simulink model "kundur_no_pss_all_methodes"  (R2023a)
settings: Solver=ode23tb  StartTime=0.0  StopTime=20  MaxStep=1/60  RelTol=1e-4  EnableMultiTasking=on
InitFcn:
  | N=200;
  | Ts=1/60;
undefined symbols (not defined in the file or in its folder): D1, Delta
libraries: spsLoadFlowBusLib x6, spsThreePhaseParallelRLCLoadLib x5, spsThreePhasePISectionLineLib x4, spsSynchronousMachinepuStandardLib x4, spsThreePhaseTransformerTwoWindingsLib x4, spsDistributedParametersLineLib x3, spsThreePhaseVIMeasurementLib x2, spsSequenceAnalyzerPhasorLib x2, spsThreePhaseBreakerLib x1, spsPower3phPhasorLib x1, spspowerguiLib x1
Description:
  | Copyright 2008-2015 The MathWorks, Inc.
settings Model: ExtModeTrigMode=oneshot  Creator=MathWorks  LastModifiedBy=felixmaldonado
settings SolverCC: AlgebraicLoopSolver=TrustRegion
settings DataIOCC: SaveFormat=Array  SignalLoggingSaveFormat=ModelDataLogs  SaveOutput=off  SaveTime=off  ReturnWorkspaceOutputs=off  TimeSaveName=t  SignalLoggingName=sigsOut
settings OptimizationCC: BlockReduction=off  BooleanDataType=off  ExpressionDepthLimit=2147483647  InitFltsAndDblsToZero=on  LifeSpan=inf
settings DebuggingCC: UnderspecifiedInitializationDetection=Classic  MergeDetectMultiDrivingBlocksExec=none  SignalResolutionControl=TryResolveAllWithWarning  MultiTaskDSMMsg=warning  MultiTaskCondExecSysMsg=none  FcnCallInpInsideContextMsg=warning  UnconnectedInputMsg=warning  UnconnectedLineMsg=warning  StateNameClashWarn=warning  SFUnexpectedBacktrackingDiag=warning  SFNoUnconditionalDefaultTransitionDiag=warning  SFExecutionAtInitializationDiag=none  ArithmeticOperatorsInVariantConditions=warning
settings HardwareCC: ProdBitPerPointer=32  ProdBitPerSizeT=32  ProdBitPerPtrDiffT=32  ProdLargestAtomicFloat=None  ProdIntDivRoundTo=Undefined  ProdEndianess=Unspecified  ProdWordSize=32  ProdHWDeviceType=32-bit Generic  TargetUnknown=on
settings ModelReferenceCC: PropagateSignalLabelsOutOfModel=off
settings SFSimCC: SimUseLocalCustomCode=off  CustomCodeUndefinedFunction=UseInterfaceOnly
settings RTWCC: RTWUseLocalCustomCode=off
settings CodeAppCC: StateflowObjectComments=on
settings GRTTargetCC: TargetLangStandard=C89/C90 (ANSI)  CombineOutputUpdateFcns=off  GRTInterface=on
settings ConfigComp: CovMetricSettings=dw  CovSaveCumulativeToWorkspaceVar=on  CovSaveSingleToWorkspaceVar=on  CovExternalEMLEnable=off  CovSFcnEnable=off
settings SimscapeCC: SimscapeNormalizeSystem=off

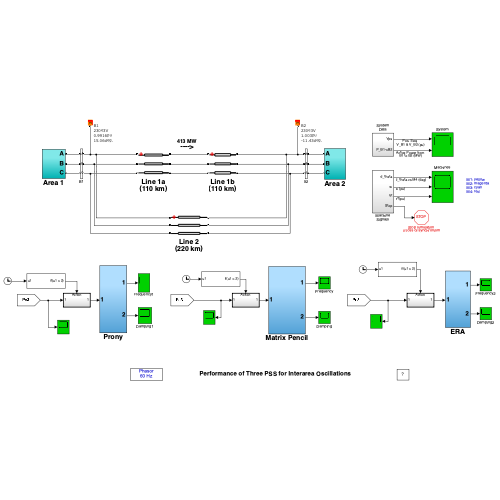
[thumbnail: Simulink's stored preview of the top-level diagram]
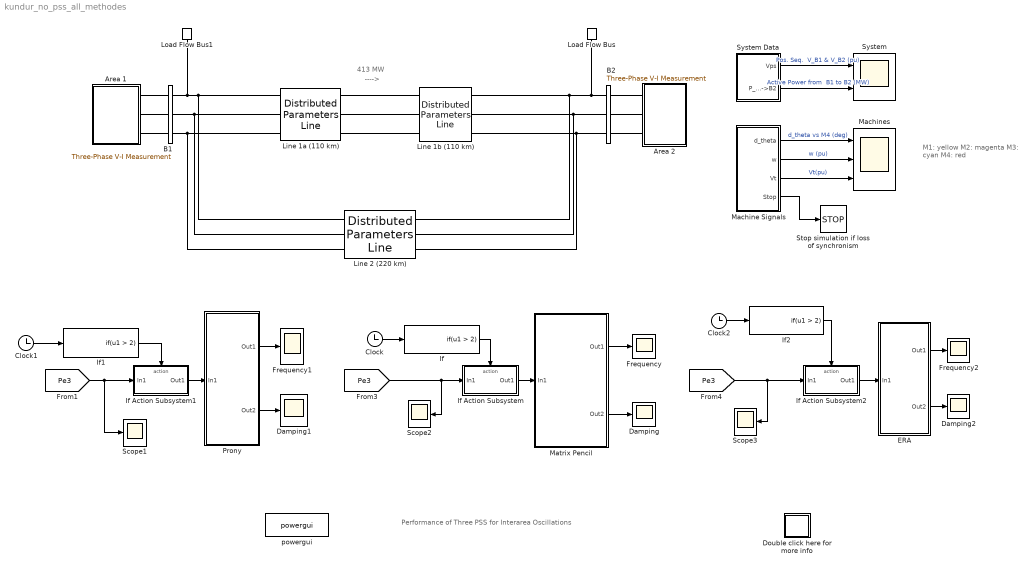
== system kundur_no_pss_all_methodes ==
  note: Performance of Three PSS for Interarea Oscillations
  note: M1: yellow
      | M2: magenta
      | M3: cyan
      | M4: red
  note: ---->
  note: 413 MW
  Area 1 : Subsystem
  Area 2 : Subsystem
  B1 : spsThreePhaseVIMeasurementLib/Three-Phase V-I Measurement  VoltageMeasurement=phase-to-ground  SetLabelV=on  LabelV=Vabc_B1  Vpu=off  VpuLL=off  CurrentMeasurement=yes  SetLabelI=on  LabelI=Iabc_B1  Ipu=off  Pbase=100e6  Vbase=500e3  OutputType=Complex  PhasorSimulation=on  PSBequivalent=0
  B2 : spsThreePhaseVIMeasurementLib/Three-Phase V-I Measurement  VoltageMeasurement=phase-to-ground  SetLabelV=on  LabelV=Vabc_B2  Vpu=off  VpuLL=off  CurrentMeasurement=yes  SetLabelI=on  LabelI=Iabc_B2  Ipu=off  Pbase=100e6  Vbase=500e3  OutputType=Complex  PhasorSimulation=on  PSBequivalent=0
  Clock : Clock
  Clock1 : Clock
  Clock2 : Clock
  Damping : Scope
  Damping1 : Scope
  Damping2 : Scope
  Double click here for more info : Subsystem
      settings: OpenFcn=showdemo(bdroot(gcb))
      mask Display: disp('?')
  ERA : Subsystem
  Frequency : Scope
  Frequency1 : Scope
  Frequency2 : Scope
  If : If  IfExpression=u1 > 2  ShowElse=off
  If Action Subsystem : Subsystem  TreatAsAtomicUnit=on
  If Action Subsystem1 : Subsystem  TreatAsAtomicUnit=on
  If Action Subsystem2 : Subsystem  TreatAsAtomicUnit=on
  If1 : If  IfExpression=u1 > 2  ShowElse=off
  If2 : If  IfExpression=u1 > 2  ShowElse=off
  Line 1a (110 km) : spsDistributedParametersLineLib/Distributed Parameters Line  Phases=3  Length=110  Frequency=60  Resistance=[0.0001*529 1.61]  Inductance=[0.001*529/(377) 0.0061]  Capacitance=[0.00175/529/(377) 5.2489e-9]  x1=[3.8639158388023e-08 228065.282846779 228065.232417196;376.991118430775 376.991118430775 376.991118430775;-0.600540727316574 0.641001708190165 -0.929792189501776]  x2=[2.61662140985057e-08 225633.072942765 225632.837043247;376.991118430775 376.991118430775 376.991118430775;-0.986420545168886 0.407422059296571 -1.16337164754703]  x3=[2.2632718889879e-11 336.03871645381 336.037634042508;376.991118430775 376.991118430775 376.991118430775;1.8256601366186 -2.54731502272154 2.16506718382181]  x4=[7.36776449333454e-11 1450.99138096572 1450.98995609566;376.991118430775 376.991118430775 376.991118430775;-1.01301435290975 0.484705984236178 -1.08608998759577]  x5=0.000622431770558027  V1=ones(3,3)  V2=ones(3,3)  I1=ones(3,3)  I2=ones(3,3)  nHarmo=1  Measurements=None  Decoupling=off  VsMag0=0  VrMag0=0  VsAngle0=0  VrAngle0=0  IsMag0=0  IrMag0=0  IsAngle0=0  IrAngle0=0
      settings: AttributesFormatString=\n  LibrarySourceBlock=sps_lib/Power Grid Elements/Distributed Parameters Line
  Line 1b (110 km) : spsDistributedParametersLineLib/Distributed Parameters Line  Phases=3  Length=110  Frequency=60  Resistance=[0.0001*529 1.61]  Inductance=[0.001*529/(377) 0.0061]  Capacitance=[0.00175/529/(377) 5.2489e-9]  x1=[2.61662140985057e-08 225633.072942765 225632.837043247;376.991118430775 376.991118430775 376.991118430775;-0.986420545168886 0.407422059296571 -1.16337164754703]  x2=[1.96331439687636e-08 230635.983486102 230635.554670201;376.991118430775 376.991118430775 376.991118430775;-1.70223885434449 0.178613473681849 -1.39218042790549]  x3=[2.98939585655011e-11 348.890847759972 348.889760478068;376.991118430775 376.991118430775 376.991118430775;2.05678749014555 -2.40728630159656 2.30509610560278]  x4=[6.51521319057991e-11 1438.08029667253 1438.07888403635;376.991118430775 376.991118430775 376.991118430775;-1.27922422756789 0.338636937194732 -1.2321590219245]  x5=0.000622431770558027  V1=ones(3,3)  V2=ones(3,3)  I1=ones(3,3)  I2=ones(3,3)  nHarmo=1  Measurements=None  Decoupling=off  VsMag0=0  VrMag0=0  VsAngle0=0  VrAngle0=0  IsMag0=0  IrMag0=0  IsAngle0=0  IrAngle0=0
      settings: AttributesFormatString=\n  LibrarySourceBlock=sps_lib/Power Grid Elements/Distributed Parameters Line
  Line 2 (220 km) : spsDistributedParametersLineLib/Distributed Parameters Line  Phases=3  Length=220  Frequency=60  Resistance=[0.0001*529 1.61]  Inductance=[0.001*529/(377) 0.0061]  Capacitance=[0.00175/529/(377) 5.2489e-9]  x1=[3.8639158388023e-08 228065.282846779 228065.232417196;376.991118430775 376.991118430775 376.991118430775;-0.835191976646093 0.49548881423357 -1.07530508345837]  x2=[1.96331439687636e-08 230635.983486102 230635.554670201;376.991118430775 376.991118430775 376.991118430775;-1.936890103674 0.0331005797252549 -1.53769332186209]  x3=[2.18539779503067e-11 335.641578515064 335.640503974824;376.991118430775 376.991118430775 376.991118430775;1.57451462094119 -2.69325063508951 2.01913162677061]  x4=[5.95777091396547e-11 1425.67040358948 1425.6690039208;376.991118430775 376.991118430775 376.991118430775;-1.49093562018794 0.193193498573398 -1.37760246372871]  x5=0.00124486354111605  V1=ones(3,3)  V2=ones(3,3)  I1=ones(3,3)  I2=ones(3,3)  nHarmo=1  Measurements=None  Decoupling=off  VsMag0=0  VrMag0=0  VsAngle0=0  VrAngle0=0  IsMag0=0  IrMag0=0  IsAngle0=0  IrAngle0=0
      settings: AttributesFormatString=\n  LibrarySourceBlock=sps_lib/Power Grid Elements/Distributed Parameters Line
  Load Flow Bus : spsLoadFlowBusLib/Load Flow Bus  LConnTagsString=a  Phases=single  Connectors=on one side  ID=B2  Vbase=230e3  Vref=1  Vangle=0  VLF=1.003  VLFb=1  VLFc=1  angleLF=-11.43  angleLFb=0  angleLFc=0
      settings: AttributesFormatString=%<ID>\n%<Vbase>V\n%<VLF>pu\n%<angleLF>deg.
  Load Flow Bus1 : spsLoadFlowBusLib/Load Flow Bus  LConnTagsString=a  Phases=single  Connectors=on one side  ID=B1  Vbase=230e3  Vref=1  Vangle=0  VLF=0.9916  VLFb=1  VLFc=1  angleLF=15.06  angleLFb=0  angleLFc=0
      settings: AttributesFormatString=%<ID>\n%<Vbase>V\n%<VLF>pu\n%<angleLF>deg.
  Machine Signals : Subsystem
  Machines : Scope  NumInputPorts=3
  Matrix Pencil : Subsystem
  Prony : Subsystem
  Scope1 : Scope
  Scope2 : Scope
  Scope3 : Scope
  Stop simulation if loss of synchronism : Stop
  System : Scope  NumInputPorts=2
  System Data : Subsystem
  powergui : spspowerguiLib/powergui  Priority=2  SimulationMode=Phasor  SampleTime=0  frequency=60  Iterations=50  frequencyindice=60  Pbase=100e6  ErrMax=0.0001  UnitsV=kV  UnitsW=MW  buscounter=0  FunctionMessages=off  echomessages=on  EnableUseOfTLC=off  CurrentSourceSwitches=off  DisableSnubberDevices=off  DisableRonSwitches=off  DisableVfSwitches=off  DisplayEquations=off  AutomaticDiscreteSolvers=off  SolverType=Tustin  Interpol=off  ExternalGateDelay=off  methode=off  Ts=0  x0status=steady  SPID=off  SwTol=0  HookPort=off  NonlinearTolerance=1e-4  nMaxIteration=100  ContinueOnMaxIteration=off  RestoreLinks=warning  ResistiveCurrentMeasurement=off  Frange=logspace(0,3,50)  Ylog=off  Xlog=off  ShowGrid=off  save=off  variable=ZData  structure=0  ZoomFFT=on  StartTime=0.0  cycles=1  DisplayStyle=1  fundamental=60  FreqAxis=off  MaxFrequency=1000  frequencyindicesteady=1  RmsSteady=1  display=off
  wires:
  Machine Signals/1(d_theta) -> Machines/1  "d_theta vs M4 (deg)"
  Machine Signals/2(w) -> Machines/2  "w (pu)"
  Machine Signals/3(Vt) -> Machines/3  "Vt(pu)"
  Machine Signals/4(Stop) -> Stop simulation if loss of synchronism/1
  System Data/1(Vps) -> System/1  "Pos. Seq.  V_B1 & V_B2 (pu)"
  System Data/2(P_B1->B2) -> System/2  "Active Power from  B1 to B2 (MW)"
  Clock/1 -> If/1
  If/1 -> If Action Subsystem/Action
  If Action Subsystem/1(Out1) -> Matrix Pencil/1(In1)
  [Pe3] -> Scope2/1, If Action Subsystem/1(In1)
  Matrix Pencil/1(Out1) -> Frequency/1
  Matrix Pencil/2(Out2) -> Damping/1
  Clock1/1 -> If1/1
  If1/1 -> If Action Subsystem1/Action
  If Action Subsystem1/1(Out1) -> Prony/1(In1)
  Prony/1(Out1) -> Frequency1/1
  Prony/2(Out2) -> Damping1/1
  [Pe3] -> Scope1/1, If Action Subsystem1/1(In1)
  Clock2/1 -> If2/1
  If2/1 -> If Action Subsystem2/Action
  If Action Subsystem2/1(Out1) -> ERA/1(In1)
  [Pe3] -> Scope3/1, If Action Subsystem2/1(In1)
  ERA/1(Out1) -> Frequency2/1
  ERA/2(Out2) -> Damping2/1
  connections:
  B1/RConn1 -- Line 1a (110 km)/LConn1 -- Line 2 (220 km)/LConn1 -- Load Flow Bus1/LConn1
  B1/RConn3 -- Line 1a (110 km)/LConn3 -- Line 2 (220 km)/LConn3
  Line 1b (110 km)/LConn1 -- Line 1a (110 km)/RConn1
  Line 1b (110 km)/LConn2 -- Line 1a (110 km)/RConn2
  Line 1a (110 km)/RConn3 -- Line 1b (110 km)/LConn3
  B2/LConn2 -- Line 1b (110 km)/RConn2 -- Line 2 (220 km)/RConn2
  Area 1/RConn2 -- B1/LConn2
  Area 1/RConn1 -- B1/LConn1
  Area 1/RConn3 -- B1/LConn3
  B1/RConn2 -- Line 1a (110 km)/LConn2 -- Line 2 (220 km)/LConn2
  B2/RConn2 -- Area 2/LConn2
  B2/RConn1 -- Area 2/LConn1
  B2/RConn3 -- Area 2/LConn3
  B2/LConn1 -- Line 1b (110 km)/RConn1 -- Line 2 (220 km)/RConn1 -- Load Flow Bus/LConn1
  B2/LConn3 -- Line 1b (110 km)/RConn3 -- Line 2 (220 km)/RConn3

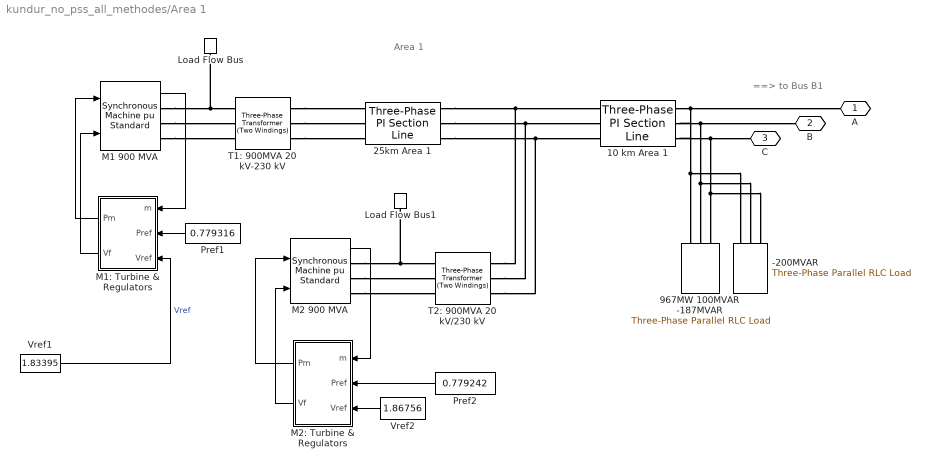
== system kundur_no_pss_all_methodes/Area 1 ==
  note: Area 1
  note: ==> to Bus B1
  -200MVAR : spsThreePhaseParallelRLCLoadLib/Three-Phase Parallel RLC Load  LConnTagsString=A|B|C  Configuration=Y (grounded)  NominalVoltage=230e3  Vabc=[1e3 1e3 1e3]  Vabcp=[1e3 1e3 1e3]  NominalFrequency=60  UnbalancedPower=off  ActivePower=0  InductivePower=0  CapacitivePower=200e6  Pabc=[10e3 9e3 11e3]  QLabc=[100 90 110]  QCabc=[100 90 110]  Pabcp=[10e3 9e3 11e3]  QLabcp=[100 90 110]  QCabcp=[100 90 110]  Measurements=None  LoadType=constant Z
  10 km Area 1 : spsThreePhasePISectionLineLib/Three-Phase PI Section Line  LConnTagsString=a|b|c  RConnTagsString=A|B|C  Length=10  Frequency=60  Resistances=[0.0001*529 1.61]  Inductances=[0.001*529/(377) 0.0061]  Capacitances=[0.00175/529/(377) 5.2489e-9]
  25km Area 1 : spsThreePhasePISectionLineLib/Three-Phase PI Section Line  LConnTagsString=a|b|c  RConnTagsString=A|B|C  Length=25  Frequency=60  Resistances=[0.0001*529 1.61]  Inductances=[0.001*529/(377) 0.0061]  Capacitances=[0.00175/529/(377) 5.2489e-9]
  967MW 100MVAR -187MVAR : spsThreePhaseParallelRLCLoadLib/Three-Phase Parallel RLC Load  LConnTagsString=A|B|C  Configuration=Y (grounded)  NominalVoltage=230e3  Vabc=[1e3 1e3 1e3]  Vabcp=[1e3 1e3 1e3]  NominalFrequency=60  UnbalancedPower=off  ActivePower=967000000  InductivePower=100e6  CapacitivePower=187e6  Pabc=[10e3 9e3 11e3]  QLabc=[100 90 110]  QCabc=[100 90 110]  Pabcp=[10e3 9e3 11e3]  QLabcp=[100 90 110]  QCabcp=[100 90 110]  Measurements=None  LoadType=constant Z
  Load Flow Bus : spsLoadFlowBusLib/Load Flow Bus  LConnTagsString=a  Phases=single  Connectors=on one side  ID=M1_Area1  Vbase=20e3  Vref=1  Vangle=0  VLF=1  VLFb=1  VLFc=1  angleLF=10.22  angleLFb=0  angleLFc=0
      settings: AttributesFormatString=%<ID>\n%<Vbase>V\n%<VLF>pu\n%<angleLF>deg.
  Load Flow Bus1 : spsLoadFlowBusLib/Load Flow Bus  LConnTagsString=a  Phases=single  Connectors=on one side  ID=M2_Area1  Vbase=20e3  Vref=1  Vangle=0  VLF=1  VLFb=1  VLFc=1  angleLF=0  angleLFb=0  angleLFc=0
      settings: AttributesFormatString=%<ID>\n%<Vbase>V\n%<VLF>pu\n%<angleLF>deg.
  M1 900 MVA : spsSynchronousMachinepuStandardLib/Synchronous Machine pu Standard  PresetModel=No  MechanicalLoad=Mechanical power Pm  ShowDetailedParameters=on  RotorType=Round  Units=per unit standard parameters  MeasurementBus=off  NominalParameters="[900E6  20000   60 ]"  Reactances1=[1.8 .3 .25 1.7 .55 .25 .2]  Reactances2=[ 1.305, 0.296, 0.252, 0.474, 0.243, 0.18 ]  dAxisTimeConstants=Open-circuit  qAxisTimeConstants=Open-circuit  TimeConstants1=[]  TimeConstants2=[8 .03 .4 .05]  TimeConstants3=[]  TimeConstants4=[]  TimeConstants5=[ 1.01, 0.053, 0.1 ]  TimeConstants6=[]  TimeConstants7=[]  TimeConstants8=[]  StatorResistance=0.0025  Mechanical=[ 6.5 0 4]  PolePairs=4  InitialConditions=[0 -31.4247 0.784454 0.784454 0.784454 2.74005 -117.26 122.74 1.83395]  SetSaturation=off  Saturation=[0.6404,0.7127,0.8441,0.9214,0.9956,1.082,1.19,1.316,1.457;0.7,0.7698,0.8872,0.9466,0.9969,1.046,1.1,1.151,1.201]  LoadFlowParameters=[1 700000000 0 0 0]  TsPowergui=0  TsBlock=-1  IterativeModel=Trapezoidal non iterative  IterativeDiscreteModel=Trapezoidal non iterative  BusType=PV  Pref=700000000  Qref=0  Qmin=-Inf  Qmax=Inf  PLF=0  QLF=0
  M1: Turbine & Regulators : Subsystem
  M2 900 MVA : spsSynchronousMachinepuStandardLib/Synchronous Machine pu Standard  PresetModel=No  MechanicalLoad=Mechanical power Pm  ShowDetailedParameters=on  RotorType=Round  Units=per unit standard parameters  MeasurementBus=off  NominalParameters="[900E6  20000   60 ]"  Reactances1=[1.8 .3 .25 1.7 .55 .25 .2]  Reactances2=[ 1.305, 0.296, 0.252, 0.474, 0.243, 0.18 ]  dAxisTimeConstants=Open-circuit  qAxisTimeConstants=Open-circuit  TimeConstants1=[]  TimeConstants2=[8 .03 .4 .05]  TimeConstants3=[]  TimeConstants4=[]  TimeConstants5=[ 1.01, 0.053, 0.1 ]  TimeConstants6=[]  TimeConstants7=[]  TimeConstants8=[]  StatorResistance=0.0025  Mechanical=[ 6.5 0 4]  PolePairs=4  InitialConditions=[0 -42.8076 0.788607 0.788607 0.788607 -9.54588 -129.546 110.454 1.86756]  SetSaturation=off  Saturation=[0.6404,0.7127,0.8441,0.9214,0.9956,1.082,1.19,1.316,1.457;0.7,0.7698,0.8872,0.9466,0.9969,1.046,1.1,1.151,1.201]  LoadFlowParameters=[2 700000000 0 0 0]  TsPowergui=0  TsBlock=-1  IterativeModel=Trapezoidal non iterative  IterativeDiscreteModel=Trapezoidal non iterative  BusType=swing  Pref=0  Qref=0  Qmin=-Inf  Qmax=Inf  PLF=0  QLF=0
  M2: Turbine & Regulators : Subsystem
  Pref1 : Constant  Value=0.779316
  Pref2 : Constant  Value=0.779242
  T1: 900MVA 20 kV-230 kV : spsThreePhaseTransformerTwoWindingsLib/Three-Phase Transformer (Two Windings)  Winding1Connection=Delta (D1)  Winding2Connection=Yg  CoreType=Three single-phase transformers  SetSaturation=off  Hysteresis=off  DataFile='hysteresis'  SetInitialFlux=off  Measurements=None  UNITS=pu  NominalPower="[ 900e6   60 ]"  Winding1="[ 20e3  1e-6   0  ]"  Winding2="[ 230e3  1e-6   0.15 ]"  Rm=500  Lm=500  L0=0.5  Saturation="[ 0,0  ;  0.005,1.2  ;  1.0,1.4 ]"  InitialFluxes=[ 0.8 , -0.8 , 0.7 ]  BreakLoop=off  DiscreteSolver=Trapezoidal iterative  DataType=off  TransfoNumber=0
  T2: 900MVA 20 kV/230 kV : spsThreePhaseTransformerTwoWindingsLib/Three-Phase Transformer (Two Windings)  Winding1Connection=Delta (D1)  Winding2Connection=Yg  CoreType=Three single-phase transformers  SetSaturation=off  Hysteresis=off  DataFile='hysteresis'  SetInitialFlux=off  Measurements=None  UNITS=pu  NominalPower=[ 900e6 60 ]  Winding1="[ 20e3 1e-6  0.0]"  Winding2=[ 230e3 1e-6 0.15]  Rm=500  Lm=500  L0=0.5  Saturation="[ 0,0  ;  0.005,1.2  ;  1.0,1.4 ]"  InitialFluxes=[ 0.8 , -0.8 , 0.7 ]  BreakLoop=off  DiscreteSolver=Trapezoidal iterative  DataType=off  TransfoNumber=0
  Vref1 : Constant  Value=1.83395
  Vref2 : Constant  Value=1.86756
  " A" : PMIOPort  Side=Right
  " B" : PMIOPort  Port=2  Side=Right
  " C" : PMIOPort  Port=3  Side=Right
  wires:
  Pref1/1 -> M1: Turbine & Regulators/2(Pref)
  Vref1/1 -> M1: Turbine & Regulators/3(Vref)  "Vref"
  Pref2/1 -> M2: Turbine & Regulators/2(Pref)
  Vref2/1 -> M2: Turbine & Regulators/3(Vref)
  M2 900 MVA/1 -> M2: Turbine & Regulators/1(m)
  M2: Turbine & Regulators/1(Pm) -> M2 900 MVA/1
  M2: Turbine & Regulators/2(Vf) -> M2 900 MVA/2
  M1: Turbine & Regulators/1(Pm) -> M1 900 MVA/1
  M1: Turbine & Regulators/2(Vf) -> M1 900 MVA/2
  M1 900 MVA/1 -> M1: Turbine & Regulators/1(m)
  connections:
  T1: 900MVA 20 kV-230 kV/RConn1 -- 25km Area 1/LConn1
  T1: 900MVA 20 kV-230 kV/RConn2 -- 25km Area 1/LConn2
  M2 900 MVA/RConn1 -- T2: 900MVA 20 kV/230 kV/LConn1 -- Load Flow Bus1/LConn1
  M2 900 MVA/RConn2 -- T2: 900MVA 20 kV/230 kV/LConn2
  M2 900 MVA/RConn3 -- T2: 900MVA 20 kV/230 kV/LConn3
  T1: 900MVA 20 kV-230 kV/RConn3 -- 25km Area 1/LConn3
  10 km Area 1/RConn1 -- " A"/RConn1 -- 967MW 100MVAR -187MVAR/LConn1 -- -200MVAR/LConn1
  10 km Area 1/RConn2 -- " B"/RConn1 -- 967MW 100MVAR -187MVAR/LConn2 -- -200MVAR/LConn2
  10 km Area 1/RConn3 -- " C"/RConn1 -- 967MW 100MVAR -187MVAR/LConn3 -- -200MVAR/LConn3
  M1 900 MVA/RConn1 -- T1: 900MVA 20 kV-230 kV/LConn1 -- Load Flow Bus/LConn1
  M1 900 MVA/RConn2 -- T1: 900MVA 20 kV-230 kV/LConn2
  M1 900 MVA/RConn3 -- T1: 900MVA 20 kV-230 kV/LConn3
  25km Area 1/RConn2 -- 10 km Area 1/LConn2 -- T2: 900MVA 20 kV/230 kV/RConn2
  25km Area 1/RConn1 -- 10 km Area 1/LConn1 -- T2: 900MVA 20 kV/230 kV/RConn1
  25km Area 1/RConn3 -- 10 km Area 1/LConn3 -- T2: 900MVA 20 kV/230 kV/RConn3

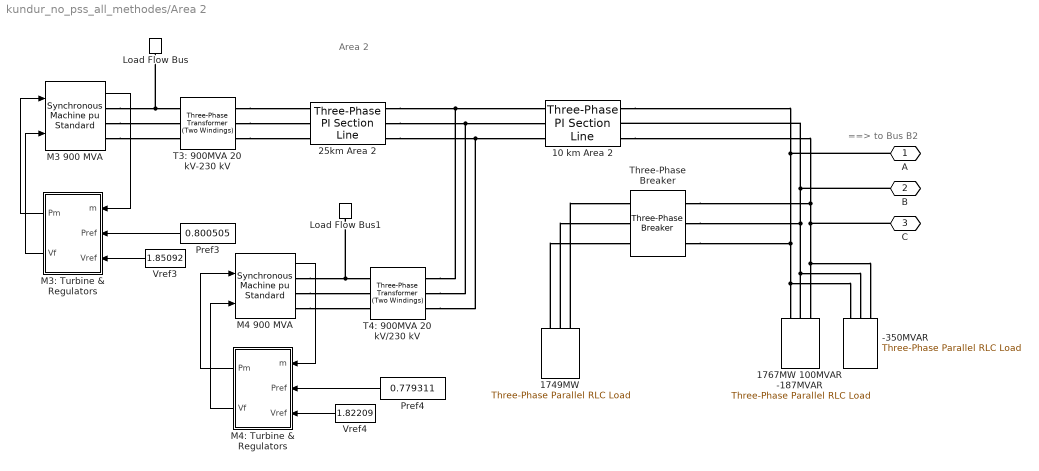
== system kundur_no_pss_all_methodes/Area 2 ==
  note: ==> to Bus B2
  note: Area 2
  -350MVAR : spsThreePhaseParallelRLCLoadLib/Three-Phase Parallel RLC Load  LConnTagsString=A|B|C  Configuration=Y (grounded)  NominalVoltage=230e3  Vabc=[1e3 1e3 1e3]  Vabcp=[1e3 1e3 1e3]  NominalFrequency=60  UnbalancedPower=off  ActivePower=0  InductivePower=0  CapacitivePower=350e6  Pabc=[10e3 9e3 11e3]  QLabc=[100 90 110]  QCabc=[100 90 110]  Pabcp=[10e3 9e3 11e3]  QLabcp=[100 90 110]  QCabcp=[100 90 110]  Measurements=None  LoadType=constant Z
  10 km Area 2 : spsThreePhasePISectionLineLib/Three-Phase PI Section Line  LConnTagsString=a|b|c  RConnTagsString=A|B|C  Length=10  Frequency=60  Resistances=[0.0001*529 1.61]  Inductances=[0.001*529/(377) 0.0061]  Capacitances=[0.00175/529/(377) 5.2489e-9]
  "1749MW " : spsThreePhaseParallelRLCLoadLib/Three-Phase Parallel RLC Load  LConnTagsString=A|B|C  Configuration=Y (grounded)  NominalVoltage=230e3  Vabc=[1e3 1e3 1e3]  Vabcp=[1e3 1e3 1e3]  NominalFrequency=60  UnbalancedPower=off  ActivePower=1749330000  InductivePower=0  CapacitivePower=0  Pabc=[10e3 9e3 11e3]  QLabc=[100 90 110]  QCabc=[100 90 110]  Pabcp=[10e3 9e3 11e3]  QLabcp=[100 90 110]  QCabcp=[100 90 110]  Measurements=None  LoadType=constant Z
  1767MW 100MVAR -187MVAR : spsThreePhaseParallelRLCLoadLib/Three-Phase Parallel RLC Load  LConnTagsString=A|B|C  Configuration=Y (grounded)  NominalVoltage=230e3  Vabc=[1e3 1e3 1e3]  Vabcp=[1e3 1e3 1e3]  NominalFrequency=60  UnbalancedPower=off  ActivePower=1767000000  InductivePower=100e6  CapacitivePower=187e6  Pabc=[10e3 9e3 11e3]  QLabc=[100 90 110]  QCabc=[100 90 110]  Pabcp=[10e3 9e3 11e3]  QLabcp=[100 90 110]  QCabcp=[100 90 110]  Measurements=None  LoadType=constant Z
  25km Area 2 : spsThreePhasePISectionLineLib/Three-Phase PI Section Line  LConnTagsString=a|b|c  RConnTagsString=A|B|C  Length=25  Frequency=60  Resistances=[0.0001*529 1.61]  Inductances=[0.001*529/(377) 0.0061]  Capacitances=[0.00175/529/(377) 5.2489e-9]
  Load Flow Bus : spsLoadFlowBusLib/Load Flow Bus  LConnTagsString=a  Phases=single  Connectors=on one side  ID=M3_Area2  Vbase=20e3  Vref=1  Vangle=0  VLF=1  VLFb=1  VLFc=1  angleLF=-15.88  angleLFb=0  angleLFc=0
      settings: AttributesFormatString=%<ID>\n%<Vbase>V\n%<VLF>pu\n%<angleLF>deg.
  Load Flow Bus1 : spsLoadFlowBusLib/Load Flow Bus  LConnTagsString=a  Phases=single  Connectors=on one side  ID=M4_Area2  Vbase=20e3  Vref=1  Vangle=0  VLF=1  VLFb=1  VLFc=1  angleLF=-26.53  angleLFb=0  angleLFc=0
      settings: AttributesFormatString=%<ID>\n%<Vbase>V\n%<VLF>pu\n%<angleLF>deg.
  M3 900 MVA : spsSynchronousMachinepuStandardLib/Synchronous Machine pu Standard  PresetModel=No  MechanicalLoad=Mechanical power Pm  ShowDetailedParameters=on  RotorType=Round  Units=per unit standard parameters  MeasurementBus=off  NominalParameters="[900E6  20000   60 ]"  Reactances1=[1.8 .3 .25 1.7 .55 .25 .2]  Reactances2=[ 1.305, 0.296, 0.252, 0.474, 0.243, 0.18 ]  dAxisTimeConstants=Open-circuit  qAxisTimeConstants=Open-circuit  TimeConstants1=[]  TimeConstants2=[8 .03 .4 .05]  TimeConstants3=[]  TimeConstants4=[]  TimeConstants5=[ 1.01, 0.053, 0.1 ]  TimeConstants6=[]  TimeConstants7=[]  TimeConstants8=[]  StatorResistance=0.0025  Mechanical=[ 6.175 0 4]  PolePairs=4  InitialConditions=[0 -56.3243 0.8041 0.8041 0.8041 -22.4087 -142.409 97.5913 1.85092]  SetSaturation=off  Saturation=[0.6404,0.7127,0.8441,0.9214,0.9956,1.082,1.19,1.316,1.457;0.7,0.7698,0.8872,0.9466,0.9969,1.046,1.1,1.151,1.201]  LoadFlowParameters=[1 719000000 0 0 0]  TsPowergui=0  TsBlock=-1  IterativeModel=Trapezoidal non iterative  IterativeDiscreteModel=Trapezoidal non iterative  BusType=PV  Pref=719000000  Qref=0  Qmin=-Inf  Qmax=Inf  PLF=0  QLF=0
  M3: Turbine & Regulators : Subsystem
  M4 900 MVA : spsSynchronousMachinepuStandardLib/Synchronous Machine pu Standard  PresetModel=No  MechanicalLoad=Mechanical power Pm  ShowDetailedParameters=on  RotorType=Round  Units=per unit standard parameters  MeasurementBus=off  NominalParameters="[900E6  20000   60 ]"  Reactances1=[1.8 .3 .25 1.7 .55 .25 .2]  Reactances2=[ 1.305, 0.296, 0.252, 0.474, 0.243, 0.18 ]  dAxisTimeConstants=Open-circuit  qAxisTimeConstants=Open-circuit  TimeConstants1=[]  TimeConstants2=[8 .03 .4 .05]  TimeConstants3=[]  TimeConstants4=[]  TimeConstants5=[ 1.01, 0.053, 0.1 ]  TimeConstants6=[]  TimeConstants7=[]  TimeConstants8=[]  StatorResistance=0.0025  Mechanical=[ 6.175 0 4]  PolePairs=4  InitialConditions=[0 -67.7513 0.783185 0.783185 0.783185 -33.2679 -153.268 86.7321 1.82209]  SetSaturation=off  Saturation=[0.6404,0.7127,0.8441,0.9214,0.9956,1.082,1.19,1.316,1.457;0.7,0.7698,0.8872,0.9466,0.9969,1.046,1.1,1.151,1.201]  LoadFlowParameters=[1 700000000 0 0 0]  TsPowergui=0  TsBlock=-1  IterativeModel=Trapezoidal non iterative  IterativeDiscreteModel=Trapezoidal non iterative  BusType=PV  Pref=700000000  Qref=0  Qmin=-Inf  Qmax=Inf  PLF=0  QLF=0
  M4: Turbine & Regulators : Subsystem
  Pref3 : Constant  Value=0.800505
  Pref4 : Constant  Value=0.779311
  T3: 900MVA 20 kV-230 kV : spsThreePhaseTransformerTwoWindingsLib/Three-Phase Transformer (Two Windings)  Winding1Connection=Delta (D1)  Winding2Connection=Yg  CoreType=Three single-phase transformers  SetSaturation=off  Hysteresis=off  DataFile='hysteresis'  SetInitialFlux=off  Measurements=None  UNITS=pu  NominalPower="[ 900e6   60 ]"  Winding1="[ 20e3  1e-6   0  ]"  Winding2="[ 230e3  1e-6   0.15 ]"  Rm=500  Lm=500  L0=0.5  Saturation="[ 0,0  ;  0.005,1.2  ;  1.0,1.4 ]"  InitialFluxes=[ 0.8 , -0.8 , 0.7 ]  BreakLoop=off  DiscreteSolver=Trapezoidal iterative  DataType=off  TransfoNumber=0
  T4: 900MVA 20 kV/230 kV : spsThreePhaseTransformerTwoWindingsLib/Three-Phase Transformer (Two Windings)  Winding1Connection=Delta (D1)  Winding2Connection=Yg  CoreType=Three single-phase transformers  SetSaturation=off  Hysteresis=off  DataFile='hysteresis'  SetInitialFlux=off  Measurements=None  UNITS=pu  NominalPower=[ 900e6 60 ]  Winding1="[ 20e3 1e-6  0.0]"  Winding2=[ 230e3 1e-6 0.15]  Rm=500  Lm=500  L0=0.5  Saturation="[ 0,0  ;  0.005,1.2  ;  1.0,1.4 ]"  InitialFluxes=[ 0.8 , -0.8 , 0.7 ]  BreakLoop=off  DiscreteSolver=Trapezoidal iterative  DataType=off  TransfoNumber=0
  Three-Phase Breaker : spsThreePhaseBreakerLib/Three-Phase Breaker  InitialState=open  SwitchA=on  SwitchB=on  SwitchC=on  SwitchTimes="[1  1+3/60]"  External=off  BreakerResistance=0.01  SnubberResistance=1e6  SnubberCapacitance=inf  Measurements=None
  Vref3 : Constant  Value=1.85092
  Vref4 : Constant  Value=1.82209
  A : PMIOPort  Side=Left
  B : PMIOPort  Port=2  Side=Left
  C : PMIOPort  Port=3  Side=Left
  wires:
  Pref3/1 -> M3: Turbine & Regulators/2(Pref)
  Vref3/1 -> M3: Turbine & Regulators/3(Vref)
  Pref4/1 -> M4: Turbine & Regulators/2(Pref)
  Vref4/1 -> M4: Turbine & Regulators/3(Vref)
  M3 900 MVA/1 -> M3: Turbine & Regulators/1(m)
  M3: Turbine & Regulators/2(Vf) -> M3 900 MVA/2
  M3: Turbine & Regulators/1(Pm) -> M3 900 MVA/1
  M4: Turbine & Regulators/1(Pm) -> M4 900 MVA/1
  M4: Turbine & Regulators/2(Vf) -> M4 900 MVA/2
  M4 900 MVA/1 -> M4: Turbine & Regulators/1(m)
  connections:
  M3 900 MVA/RConn3 -- T3: 900MVA 20 kV-230 kV/LConn3
  M3 900 MVA/RConn2 -- T3: 900MVA 20 kV-230 kV/LConn2
  M3 900 MVA/RConn1 -- T3: 900MVA 20 kV-230 kV/LConn1 -- Load Flow Bus/LConn1
  T3: 900MVA 20 kV-230 kV/RConn3 -- 25km Area 2/LConn3
  M4 900 MVA/RConn3 -- T4: 900MVA 20 kV/230 kV/LConn3
  M4 900 MVA/RConn2 -- T4: 900MVA 20 kV/230 kV/LConn2
  M4 900 MVA/RConn1 -- T4: 900MVA 20 kV/230 kV/LConn1 -- Load Flow Bus1/LConn1
  T3: 900MVA 20 kV-230 kV/RConn2 -- 25km Area 2/LConn2
  T3: 900MVA 20 kV-230 kV/RConn1 -- 25km Area 2/LConn1
  25km Area 2/RConn2 -- 10 km Area 2/LConn2 -- T4: 900MVA 20 kV/230 kV/RConn2
  25km Area 2/RConn1 -- 10 km Area 2/LConn1 -- T4: 900MVA 20 kV/230 kV/RConn1
  25km Area 2/RConn3 -- 10 km Area 2/LConn3 -- T4: 900MVA 20 kV/230 kV/RConn3
  10 km Area 2/RConn1 -- 1767MW 100MVAR -187MVAR/LConn1 -- -350MVAR/LConn1 -- Three-Phase Breaker/LConn1 -- A/RConn1
  1767MW 100MVAR -187MVAR/LConn2 -- -350MVAR/LConn2 -- Three-Phase Breaker/LConn2 -- 10 km Area 2/RConn2 -- B/RConn1
  10 km Area 2/RConn3 -- 1767MW 100MVAR -187MVAR/LConn3 -- -350MVAR/LConn3 -- C/RConn1 -- Three-Phase Breaker/LConn3
  "1749MW "/LConn1 -- Three-Phase Breaker/RConn1
  "1749MW "/LConn2 -- Three-Phase Breaker/RConn2
  "1749MW "/LConn3 -- Three-Phase Breaker/RConn3

== system kundur_no_pss_all_methodes/Double click here for more info ==

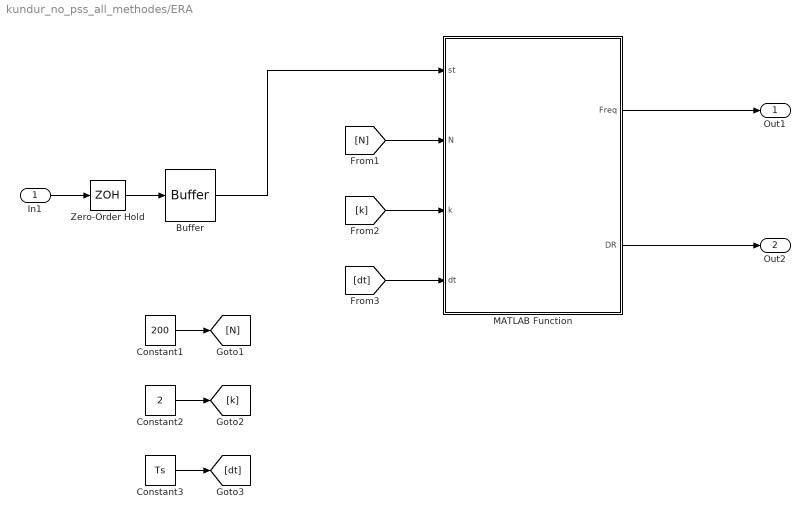
== system kundur_no_pss_all_methodes/ERA ==
  In1 : Inport
  Buffer : Buffer  N=N  V=N-1
  Constant1 : Constant  Value=200  SampleTime=Ts
  Constant2 : Constant  Value=2  SampleTime=Ts
  Constant3 : Constant  Value=Ts  SampleTime=Ts
  MATLAB Function : MATLAB Function  TreatAsAtomicUnit=on
  Zero-Order Hold : ZeroOrderHold  SampleTime=Ts
  Out1 : Outport
  Out2 : Outport  Port=2
  wires:
  [dt] -> MATLAB Function/4(dt)
  [N] -> MATLAB Function/2(N)
  Constant1/1 -> [N]
  Constant3/1 -> [dt]
  Constant2/1 -> [k]
  [k] -> MATLAB Function/3(k)
  MATLAB Function/1(Freq) -> Out1/1
  In1/1 -> Zero-Order Hold/1
  MATLAB Function/2(DR) -> Out2/1
  Buffer/1 -> MATLAB Function/1(st)
  Zero-Order Hold/1 -> Buffer/1

== system kundur_no_pss_all_methodes/If Action Subsystem ==
  In1 : Inport
  Action Port : ActionPort
  Out1 : Outport
  wires:
  In1/1 -> Out1/1

== system kundur_no_pss_all_methodes/If Action Subsystem1 ==
  In1 : Inport
  Action Port : ActionPort
  Out1 : Outport
  wires:
  In1/1 -> Out1/1

== system kundur_no_pss_all_methodes/If Action Subsystem2 ==
  In1 : Inport
  Action Port : ActionPort
  Out1 : Outport
  wires:
  In1/1 -> Out1/1

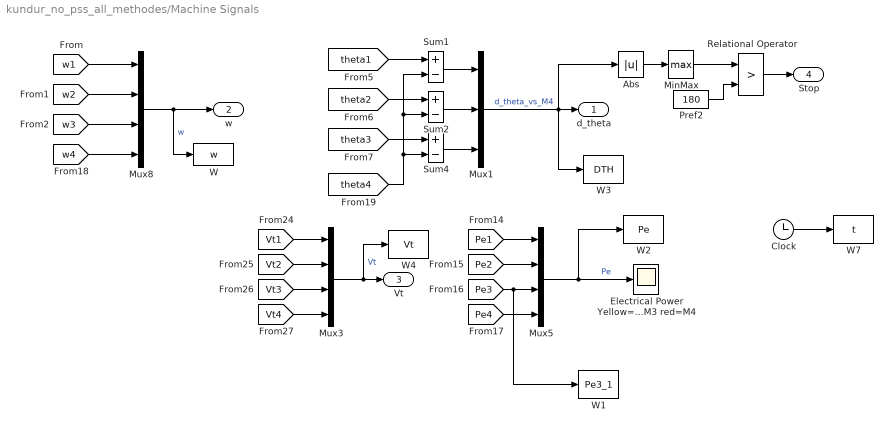
== system kundur_no_pss_all_methodes/Machine Signals ==
  Abs : Abs
  Clock : Clock
  "Electrical Power Yellow=M1 mag=M2 cyan=M3 red=M4 " : Scope
  MinMax : MinMax  Function=max  InputSameDT=on  SaturateOnIntegerOverflow=on
  Mux1 : Mux  Inputs=3
  Mux3 : Mux
  Mux5 : Mux
  Mux8 : Mux
  Pref2 : Constant  Value=180
  Relational Operator : RelationalOperator  Operator=>
  Sum1 : Sum  Inputs=+-  InputSameDT=on  SaturateOnIntegerOverflow=on  OutDataTypeStr=Inherit: Same as first input
  Sum2 : Sum  Inputs=+-  InputSameDT=on  SaturateOnIntegerOverflow=on  OutDataTypeStr=Inherit: Same as first input
  Sum4 : Sum  Inputs=+-  InputSameDT=on  SaturateOnIntegerOverflow=on  OutDataTypeStr=Inherit: Same as first input
  W : ToWorkspace  VariableName=w  SampleTime=1/60
  W1 : ToWorkspace  VariableName=Pe3_1  SampleTime=1/60
  W2 : ToWorkspace  VariableName=Pe  SampleTime=1/60
  W3 : ToWorkspace  VariableName=DTH  SampleTime=1/60
  W4 : ToWorkspace  VariableName=Vt  SampleTime=1/60
  W7 : ToWorkspace  VariableName=t  SampleTime=1/60
  d_theta : Outport
  w : Outport  Port=2
  Vt : Outport  Port=3
  Stop : Outport  Port=4
  wires:
  Mux1/1 -> d_theta/1, Abs/1, W3/1  "d_theta_vs_M4"
  Abs/1 -> MinMax/1
  Pref2/1 -> Relational Operator/2
  MinMax/1 -> Relational Operator/1
  Mux8/1 -> w/1, W/1  "w"
  Relational Operator/1 -> Stop/1
  [theta1] -> Sum1/1
  Sum1/1 -> Mux1/1
  [theta2] -> Sum2/1
  [theta3] -> Sum4/1
  [theta4] -> Sum4/2, Sum2/2, Sum1/2
  Sum2/1 -> Mux1/2
  Sum4/1 -> Mux1/3
  [Vt1] -> Mux3/1
  [Vt2] -> Mux3/2
  [Vt3] -> Mux3/3
  [Vt4] -> Mux3/4
  Mux3/1 -> Vt/1, W4/1  "Vt"
  [Pe1] -> Mux5/1
  [Pe2] -> Mux5/2
  [Pe3] -> W1/1, Mux5/3
  [Pe4] -> Mux5/4
  Mux5/1 -> "Electrical Power Yellow=M1 mag=M2 cyan=M3 red=M4 "/1, W2/1  "Pe"
  [w1] -> Mux8/1
  [w2] -> Mux8/2
  [w3] -> Mux8/3
  [w4] -> Mux8/4
  Clock/1 -> W7/1

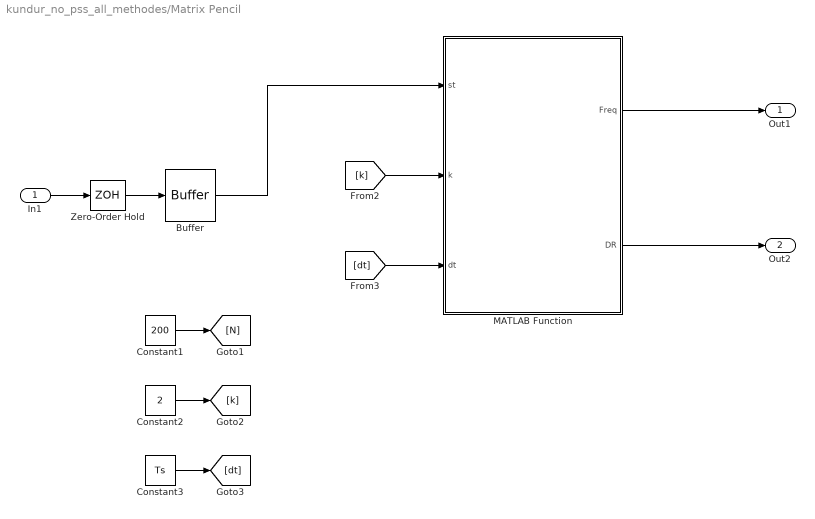
== system kundur_no_pss_all_methodes/Matrix Pencil ==
  In1 : Inport
  Buffer : Buffer  N=N  V=N-1
  Constant1 : Constant  Value=200  SampleTime=Ts
  Constant2 : Constant  Value=2  SampleTime=Ts
  Constant3 : Constant  Value=Ts  SampleTime=Ts
  MATLAB Function : MATLAB Function  TreatAsAtomicUnit=on
  Zero-Order Hold : ZeroOrderHold  SampleTime=Ts
  Out1 : Outport
  Out2 : Outport  Port=2
  wires:
  [dt] -> MATLAB Function/3(dt)
  Constant1/1 -> [N]
  Constant3/1 -> [dt]
  Constant2/1 -> [k]
  [k] -> MATLAB Function/2(k)
  MATLAB Function/1(Freq) -> Out1/1
  In1/1 -> Zero-Order Hold/1
  MATLAB Function/2(DR) -> Out2/1
  Buffer/1 -> MATLAB Function/1(st)
  Zero-Order Hold/1 -> Buffer/1

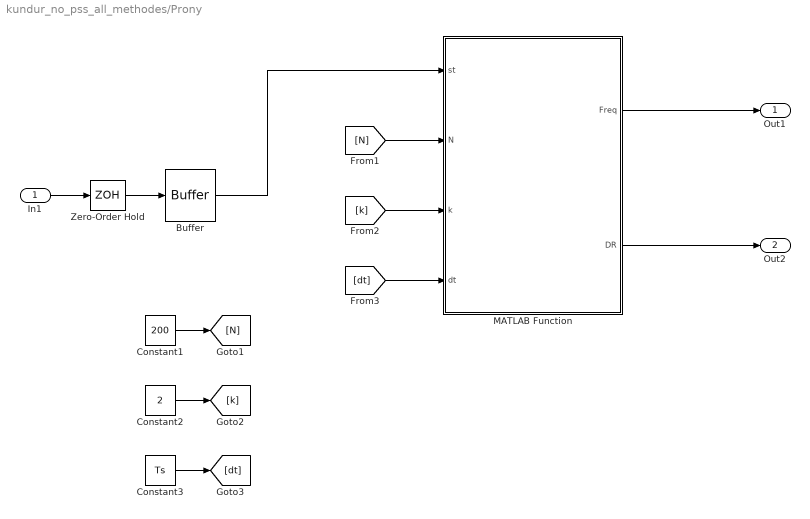
== system kundur_no_pss_all_methodes/Prony ==
  In1 : Inport
  Buffer : Buffer  N=N  V=N-1
  Constant1 : Constant  Value=200  SampleTime=Ts
  Constant2 : Constant  Value=2  SampleTime=Ts
  Constant3 : Constant  Value=Ts  SampleTime=Ts
  MATLAB Function : MATLAB Function  TreatAsAtomicUnit=on
  Zero-Order Hold : ZeroOrderHold  SampleTime=Ts
  Out1 : Outport
  Out2 : Outport  Port=2
  wires:
  [dt] -> MATLAB Function/4(dt)
  [N] -> MATLAB Function/2(N)
  Constant1/1 -> [N]
  Constant3/1 -> [dt]
  Constant2/1 -> [k]
  [k] -> MATLAB Function/3(k)
  MATLAB Function/1(Freq) -> Out1/1
  In1/1 -> Zero-Order Hold/1
  MATLAB Function/2(DR) -> Out2/1
  Buffer/1 -> MATLAB Function/1(st)
  Zero-Order Hold/1 -> Buffer/1

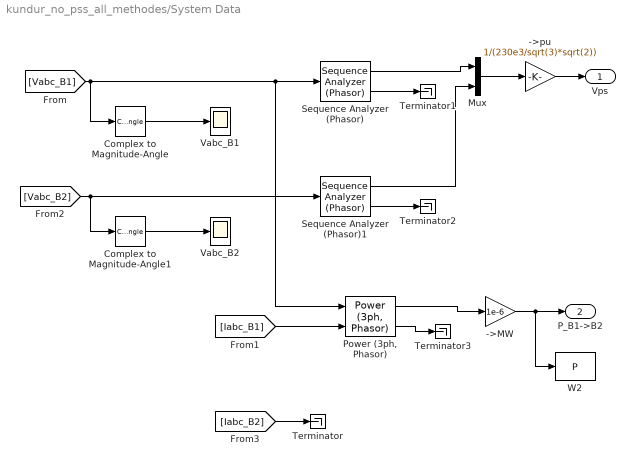
== system kundur_no_pss_all_methodes/System Data ==
  ->MW : Gain  Gain=1e-6  SaturateOnIntegerOverflow=on  OutDataTypeStr=Inherit: Same as input  ParamDataTypeStr=Inherit: Same as input
  ->pu : Gain  Gain=1/(230e3/sqrt(3)*sqrt(2))  SaturateOnIntegerOverflow=on  OutDataTypeStr=Inherit: Same as input  ParamDataTypeStr=Inherit: Same as input
  Complex to Magnitude-Angle : ComplexToMagnitudeAngle  Output=Magnitude
  Complex to Magnitude-Angle1 : ComplexToMagnitudeAngle  Output=Magnitude
  Mux : Mux  Inputs=2
  "Power (3ph, Phasor)" : spsPower3phPhasorLib/Power (3ph, Phasor)
      settings: LibrarySourceBlock=|
      | sps_lib/Sensors and Measurements/Power
      | (3ph, Phasor)
  Sequence Analyzer (Phasor) : spsSequenceAnalyzerPhasorLib/Sequence Analyzer (Phasor)  seq=Positive
      settings: LibrarySourceBlock=|
      | sps_lib/Sensors and Measurements/Sequence Analyzer
      | (Phasor)
  Sequence Analyzer (Phasor)1 : spsSequenceAnalyzerPhasorLib/Sequence Analyzer (Phasor)  seq=Positive
      settings: LibrarySourceBlock=|
      | sps_lib/Sensors and Measurements/Sequence Analyzer
      | (Phasor)
  Terminator{,1..3} (4 alike) : Terminator
  Vabc_B1 : Scope
  Vabc_B2 : Scope
  W2 : ToWorkspace  VariableName=P  SampleTime=1/60
  Vps : Outport
  P_B1->B2 : Outport  Port=2
  wires:
  [Vabc_B1] -> Sequence Analyzer (Phasor)/1, "Power (3ph, Phasor)"/1, Complex to Magnitude-Angle/1
  [Vabc_B2] -> Sequence Analyzer (Phasor)1/1, Complex to Magnitude-Angle1/1
  [Iabc_B2] -> Terminator/1
  Sequence Analyzer (Phasor)/2 -> Terminator1/1
  Sequence Analyzer (Phasor)1/2 -> Terminator2/1
  Sequence Analyzer (Phasor)1/1 -> Mux/2
  [Iabc_B1] -> "Power (3ph, Phasor)"/2
  ->pu/1 -> Vps/1
  Sequence Analyzer (Phasor)/1 -> Mux/1
  Mux/1 -> ->pu/1
  ->MW/1 -> P_B1->B2/1, W2/1
  Complex to Magnitude-Angle/1 -> Vabc_B1/1
  Complex to Magnitude-Angle1/1 -> Vabc_B2/1
  "Power (3ph, Phasor)"/1 -> ->MW/1
  "Power (3ph, Phasor)"/2 -> Terminator3/1

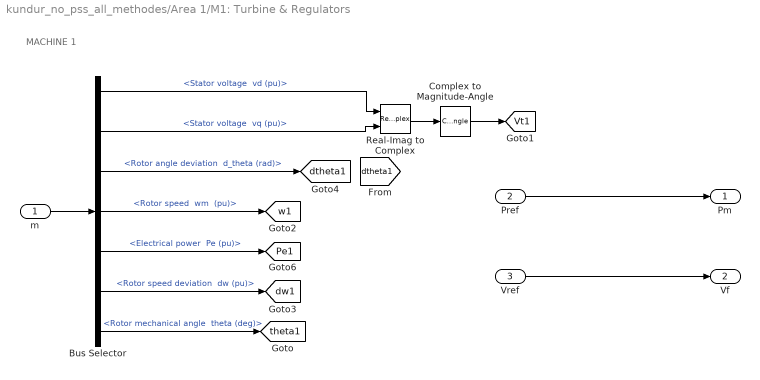
== system kundur_no_pss_all_methodes/Area 1/M1: Turbine & Regulators ==
  note: MACHINE 1
  m : Inport
  Pref : Inport  Port=2
  Vref : Inport  Port=3
  Bus Selector : BusSelector  OutputSignals="dq0 components.Stator voltage  vd (pu),dq0 components.Stator voltage  vq (pu),Mechanical.Rotor angle deviation  d_theta (rad),Mechanical.Rotor speed  wm  (pu),Mechanical.Electrical power  Pe (pu),Mechanical.Rotor speed deviation  dw (pu),Mechanical.Rotor mechanical angle  theta (deg)"
  Complex to Magnitude-Angle : ComplexToMagnitudeAngle  Output=Magnitude
  Real-Imag to Complex : RealImagToComplex
  Pm : Outport  InitialOutput=0
  Vf : Outport  Port=2  InitialOutput=0
  tag scope: Pe1=global, Vt1=global, dtheta1=global, dw1=global, theta1=global, w1=global
  wires:
  Bus Selector/1 -> Real-Imag to Complex/1  "<Stator voltage  vd (pu)>"
  Bus Selector/2 -> Real-Imag to Complex/2  "<Stator voltage  vq (pu)>"
  m/1 -> Bus Selector/1
  Real-Imag to Complex/1 -> Complex to Magnitude-Angle/1
  Vref/1 -> Vf/1
  Complex to Magnitude-Angle/1 -> [Vt1]
  Bus Selector/7 -> [theta1]  "<Rotor mechanical angle  theta (deg)>"
  Bus Selector/4 -> [w1]  "<Rotor speed  wm  (pu)>"
  Bus Selector/5 -> [Pe1]  "<Electrical power  Pe (pu)>"
  Bus Selector/6 -> [dw1]  "<Rotor speed deviation  dw (pu)>"
  Pref/1 -> Pm/1
  Bus Selector/3 -> [dtheta1]  "<Rotor angle deviation  d_theta (rad)>"

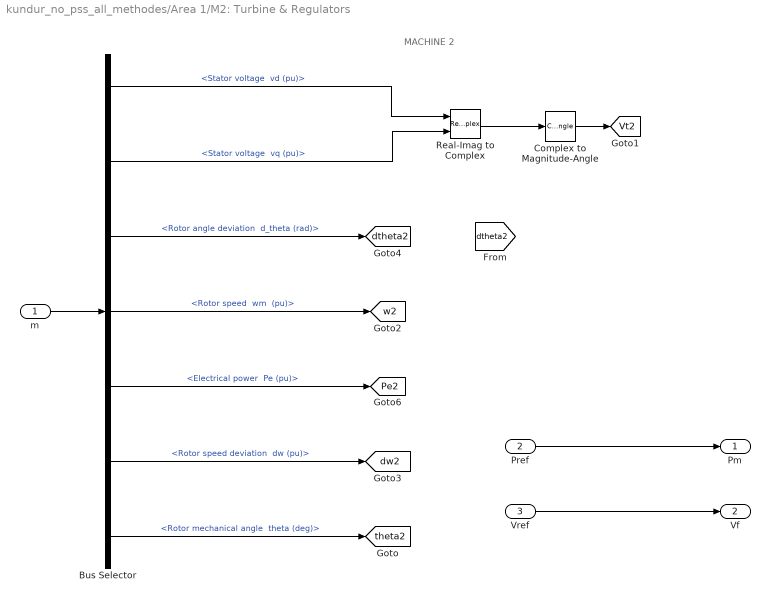
== system kundur_no_pss_all_methodes/Area 1/M2: Turbine & Regulators ==
  note: MACHINE 2
  m : Inport
  Pref : Inport  Port=2
  Vref : Inport  Port=3
  Bus Selector : BusSelector  OutputSignals="dq0 components.Stator voltage  vd (pu),dq0 components.Stator voltage  vq (pu),Mechanical.Rotor angle deviation  d_theta (rad),Mechanical.Rotor speed  wm  (pu),Mechanical.Electrical power  Pe (pu),Mechanical.Rotor speed deviation  dw (pu),Mechanical.Rotor mechanical angle  theta (deg)"
  Complex to Magnitude-Angle : ComplexToMagnitudeAngle  Output=Magnitude
  Real-Imag to Complex : RealImagToComplex
  Pm : Outport  InitialOutput=0
  Vf : Outport  Port=2  InitialOutput=0
  tag scope: Pe2=global, Vt2=global, dtheta2=global, dw2=global, theta2=global, w2=global
  wires:
  Bus Selector/6 -> [dw2]  "<Rotor speed deviation  dw (pu)>"
  Bus Selector/5 -> [Pe2]  "<Electrical power  Pe (pu)>"
  Bus Selector/4 -> [w2]  "<Rotor speed  wm  (pu)>"
  Bus Selector/7 -> [theta2]  "<Rotor mechanical angle  theta (deg)>"
  Complex to Magnitude-Angle/1 -> [Vt2]
  Vref/1 -> Vf/1
  Real-Imag to Complex/1 -> Complex to Magnitude-Angle/1
  Bus Selector/2 -> Real-Imag to Complex/2  "<Stator voltage  vq (pu)>"
  Bus Selector/1 -> Real-Imag to Complex/1  "<Stator voltage  vd (pu)>"
  Pref/1 -> Pm/1
  Bus Selector/3 -> [dtheta2]  "<Rotor angle deviation  d_theta (rad)>"
  m/1 -> Bus Selector/1

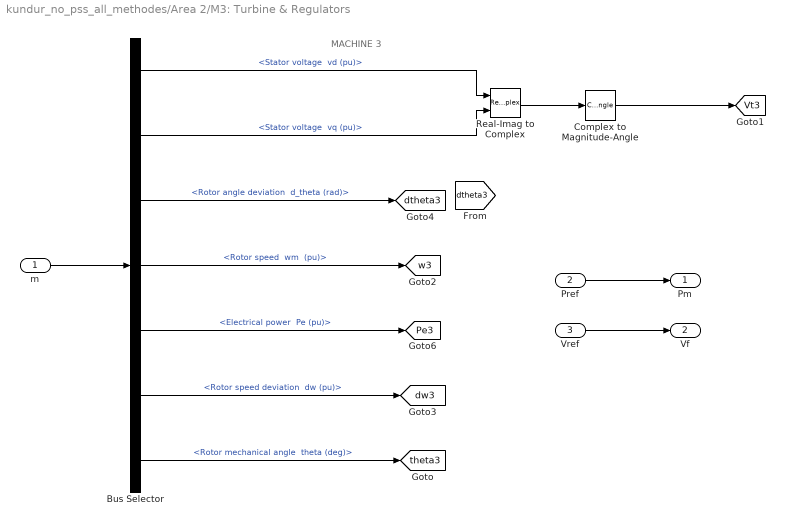
== system kundur_no_pss_all_methodes/Area 2/M3: Turbine & Regulators ==
  note: MACHINE 3
  m : Inport
  Pref : Inport  Port=2
  Vref : Inport  Port=3
  Bus Selector : BusSelector  OutputSignals="dq0 components.Stator voltage  vd (pu),dq0 components.Stator voltage  vq (pu),Mechanical.Rotor angle deviation  d_theta (rad),Mechanical.Rotor speed  wm  (pu),Mechanical.Electrical power  Pe (pu),Mechanical.Rotor speed deviation  dw (pu),Mechanical.Rotor mechanical angle  theta (deg)"
  Complex to Magnitude-Angle : ComplexToMagnitudeAngle  Output=Magnitude
  Real-Imag to Complex : RealImagToComplex
  Pm : Outport  InitialOutput=0
  Vf : Outport  Port=2  InitialOutput=0
  tag scope: Pe3=global, Vt3=global, dtheta3=global, dw3=global, theta3=global, w3=global
  wires:
  Bus Selector/6 -> [dw3]  "<Rotor speed deviation  dw (pu)>"
  Bus Selector/5 -> [Pe3]  "<Electrical power  Pe (pu)>"
  Bus Selector/4 -> [w3]  "<Rotor speed  wm  (pu)>"
  Bus Selector/7 -> [theta3]  "<Rotor mechanical angle  theta (deg)>"
  Complex to Magnitude-Angle/1 -> [Vt3]
  Vref/1 -> Vf/1
  Real-Imag to Complex/1 -> Complex to Magnitude-Angle/1
  Bus Selector/2 -> Real-Imag to Complex/2  "<Stator voltage  vq (pu)>"
  Bus Selector/1 -> Real-Imag to Complex/1  "<Stator voltage  vd (pu)>"
  Bus Selector/3 -> [dtheta3]  "<Rotor angle deviation  d_theta (rad)>"
  Pref/1 -> Pm/1
  m/1 -> Bus Selector/1

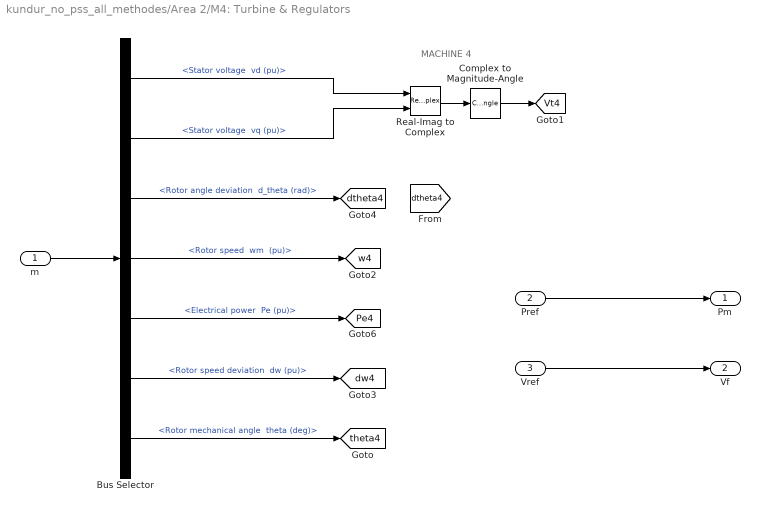
== system kundur_no_pss_all_methodes/Area 2/M4: Turbine & Regulators ==
  note: MACHINE 4
  m : Inport
  Pref : Inport  Port=2
  Vref : Inport  Port=3
  Bus Selector : BusSelector  OutputSignals="dq0 components.Stator voltage  vd (pu),dq0 components.Stator voltage  vq (pu),Mechanical.Rotor angle deviation  d_theta (rad),Mechanical.Rotor speed  wm  (pu),Mechanical.Electrical power  Pe (pu),Mechanical.Rotor speed deviation  dw (pu),Mechanical.Rotor mechanical angle  theta (deg)"
  Complex to Magnitude-Angle : ComplexToMagnitudeAngle  Output=Magnitude
  Real-Imag to Complex : RealImagToComplex
  Pm : Outport  InitialOutput=0
  Vf : Outport  Port=2  InitialOutput=0
  tag scope: Pe4=global, Vt4=global, dtheta4=global, dw4=global, theta4=global, w4=global
  wires:
  Bus Selector/1 -> Real-Imag to Complex/1  "<Stator voltage  vd (pu)>"
  Bus Selector/2 -> Real-Imag to Complex/2  "<Stator voltage  vq (pu)>"
  Pref/1 -> Pm/1
  Real-Imag to Complex/1 -> Complex to Magnitude-Angle/1
  Vref/1 -> Vf/1
  Complex to Magnitude-Angle/1 -> [Vt4]
  Bus Selector/7 -> [theta4]  "<Rotor mechanical angle  theta (deg)>"
  Bus Selector/4 -> [w4]  "<Rotor speed  wm  (pu)>"
  Bus Selector/5 -> [Pe4]  "<Electrical power  Pe (pu)>"
  Bus Selector/6 -> [dw4]  "<Rotor speed deviation  dw (pu)>"
  Bus Selector/3 -> [dtheta4]  "<Rotor angle deviation  d_theta (rad)>"
  m/1 -> Bus Selector/1

== matlab function kundur_no_pss_all_methodes/Prony/MATLAB Function ==
  data: st input; Freq output size=2; DR output size=2; N input; k input; dt input
function [Freq, DR] = prony(st, N, k, dt)
st = st - mean(st);
b = st(k+1:N,1);
b1 = st(k:N-1);
R1 = st(k:-1:1);
T = toeplitz(b1,R1);
a = pinv(T)*b;
p = [1 -1*a'];
z = roots(p);
lambda = log(z)/dt;
sigma = -real(lambda);
omega = imag(lambda);
fre1 = omega/(2*pi);
damp = sigma;
aux = [fre1 damp];
aux = sortrows(aux);
fre1 = aux(:,1);
damp = aux(:,2);
Freq = fre1((k/2)+1:k);
dr1 = damp((k/2)+1:k);
DR =(dr1./sqrt((dr1.^2)+((Freq*2*pi).^2)))*100;
end

== matlab function kundur_no_pss_all_methodes/Matrix Pencil/MATLAB Function ==
  data: st input; Freq output size=2; DR output size=2; k input; dt input
function [Freq, DR] = matrix_pencil(st, k, dt)
st = st - mean(st);
L = 100;
N = 200;
Y = zeros(N-L, N-L+1);
for i = 1:(N-L)
    Y(i,:) = st(i:(i+L));
end
[U,S,V] = svd(Y);
D = diag(S);              
Vnew = V(:,1:k);
a = size(Vnew,1);
Vs1 = Vnew(1:(a-1),:);
Vs2 = Vnew(2:end,:);
Y1 = Vs1'*Vs1;   
Y2 = Vs2'*Vs1;
Y1 = Y1';
Y1Y2 = inv(Y1)*Y2;
Y1Y2(isnan(Y1Y2)) = 0;
E = eig(Y1Y2);
lambda = log(E)/dt;
sigma = -real(lambda);
omega = imag(lambda);
fre1 = omega/(2*pi);
damp = sigma;
aux = [fre1 damp];
aux = sortrows(aux);
fre1 = aux(:,1);
damp = aux(:,2);
Freq = fre1((k/2)+1:k);
dr1 = damp((k/2)+1:k);
DR =(dr1./sqrt((dr1.^2)+((Freq*2*pi).^2)))*100;
end

== matlab function kundur_no_pss_all_methodes/ERA/MATLAB Function ==
  data: st input; Freq output size=2; DR output size=2; N input; k input; dt input
function [Freq, DR] = ERA(st, N , k, dt)
st = st - mean(st);
r = round(N/2) - 1;
H0 = hankel(st(1:r), st(r:end-2));
H1 = hankel(st(2:r+1), st(r+1:end-1));
[U,S,V] = svd(H0);
Sn = S(1:k,1:k);
Un = U(:,1:k);
Vt = V';
Vn = Vt(1:k,:);
D = sqrt(Sn);
A = D\Un'*H1*Vn'/D;
A(isnan(A)) = 0;
E = eig(A);
lambda = log(E)/dt;
sigma = -real(lambda);
omega = imag(lambda);
fre1 = omega/(2*pi);
damp = sigma;
aux = [fre1 damp];
aux = sortrows(aux);
fre1 = aux(:,1);
damp = aux(:,2);
Freq = fre1((k/2)+1:k);
dr1 = damp((k/2)+1:k);
DR =(dr1./sqrt((dr1.^2)+((Freq*2*pi).^2)))*100;
end
